simulink model "VTOL_v2"  (R2019b)
settings: Solver=FixedStepAuto  StartTime=0.0  StopTime=inf  FixedStep=Ts  RelTol=1e-3  EnableMultiTasking=on
values from neighbouring files (symbols this model uses):
  k1 = (0.5/axisgains(2) - k2*cruiseThrottle^2)/(cruiseVel^2)    [SensitivityParameterFinder.m]
  k2 = 0.5/(axisgains(2)*hoverpower(1).^2)    [SensitivityParameterFinder.m]
  k3 = (0.5/axisgains(1) - k4*cruiseThrottle^2)/(cruiseVel^2)    [SensitivityParameterFinder.m]
  k4 = 0.5/(axisgains(1)*hoverpower(1).^2)    [SensitivityParameterFinder.m]
  Ts = 1/100    (= 0.01)    [VTOL_params.m]
undefined symbols (not defined in the file or in its folder): color, deltaprops, dev, led_mask, Main, mode, MRC, pwm_output0
libraries: px4uORBlib x13, aerolibutil x8, simulink x6, pwm_sig_converters x4, px4Sensorslib x2, px4lib x2, sharedtransform x2
(part 2 of 3)

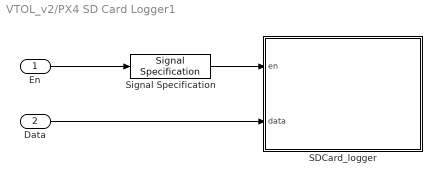
== system VTOL_v2/PX4 SD Card Logger1 ==
  En : Inport
  Data : Inport  Port=2
  SDCard_logger : MATLAB Function  TreatAsAtomicUnit=on
  Signal Specification : SignalSpecification  OutDataTypeStr=boolean
  wires:
  Signal Specification/1 -> SDCard_logger/1(en)
  En/1 -> Signal Specification/1
  Data/1 -> SDCard_logger/2(data)

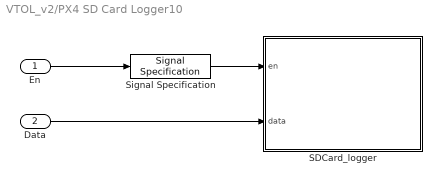
== system VTOL_v2/PX4 SD Card Logger10 ==
  En : Inport
  Data : Inport  Port=2
  SDCard_logger : MATLAB Function  TreatAsAtomicUnit=on
  Signal Specification : SignalSpecification  OutDataTypeStr=boolean
  wires:
  Signal Specification/1 -> SDCard_logger/1(en)
  En/1 -> Signal Specification/1
  Data/1 -> SDCard_logger/2(data)

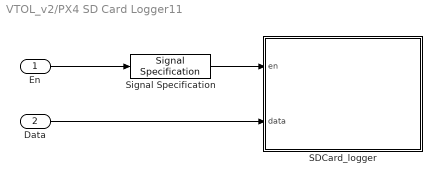
== system VTOL_v2/PX4 SD Card Logger11 ==
  En : Inport
  Data : Inport  Port=2
  SDCard_logger : MATLAB Function  TreatAsAtomicUnit=on
  Signal Specification : SignalSpecification  OutDataTypeStr=boolean
  wires:
  Signal Specification/1 -> SDCard_logger/1(en)
  En/1 -> Signal Specification/1
  Data/1 -> SDCard_logger/2(data)

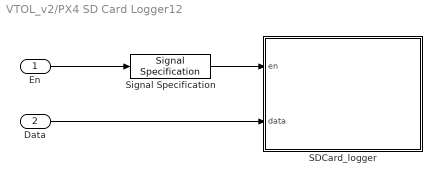
== system VTOL_v2/PX4 SD Card Logger12 ==
  En : Inport
  Data : Inport  Port=2
  SDCard_logger : MATLAB Function  TreatAsAtomicUnit=on
  Signal Specification : SignalSpecification  OutDataTypeStr=boolean
  wires:
  Signal Specification/1 -> SDCard_logger/1(en)
  En/1 -> Signal Specification/1
  Data/1 -> SDCard_logger/2(data)

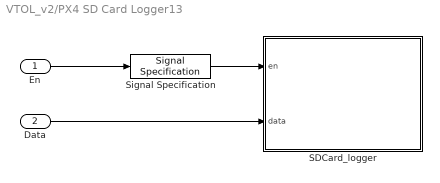
== system VTOL_v2/PX4 SD Card Logger13 ==
  En : Inport
  Data : Inport  Port=2
  SDCard_logger : MATLAB Function  TreatAsAtomicUnit=on
  Signal Specification : SignalSpecification  OutDataTypeStr=boolean
  wires:
  Signal Specification/1 -> SDCard_logger/1(en)
  En/1 -> Signal Specification/1
  Data/1 -> SDCard_logger/2(data)

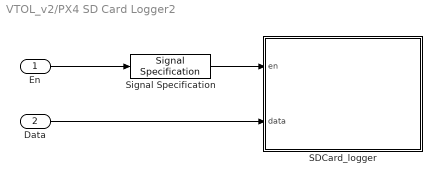
== system VTOL_v2/PX4 SD Card Logger2 ==
  En : Inport
  Data : Inport  Port=2
  SDCard_logger : MATLAB Function  TreatAsAtomicUnit=on
  Signal Specification : SignalSpecification  OutDataTypeStr=boolean
  wires:
  Signal Specification/1 -> SDCard_logger/1(en)
  En/1 -> Signal Specification/1
  Data/1 -> SDCard_logger/2(data)

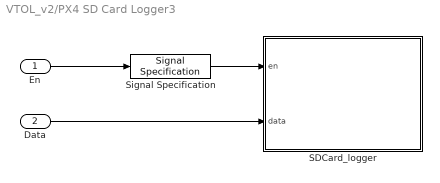
== system VTOL_v2/PX4 SD Card Logger3 ==
  En : Inport
  Data : Inport  Port=2
  SDCard_logger : MATLAB Function  TreatAsAtomicUnit=on
  Signal Specification : SignalSpecification  OutDataTypeStr=boolean
  wires:
  Signal Specification/1 -> SDCard_logger/1(en)
  En/1 -> Signal Specification/1
  Data/1 -> SDCard_logger/2(data)

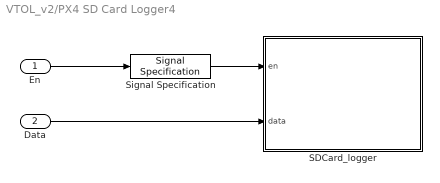
== system VTOL_v2/PX4 SD Card Logger4 ==
  En : Inport
  Data : Inport  Port=2
  SDCard_logger : MATLAB Function  TreatAsAtomicUnit=on
  Signal Specification : SignalSpecification  OutDataTypeStr=boolean
  wires:
  Signal Specification/1 -> SDCard_logger/1(en)
  En/1 -> Signal Specification/1
  Data/1 -> SDCard_logger/2(data)

== system VTOL_v2/PX4 SD Card Logger5 ==
  En : Inport
  Data : Inport  Port=2
  SDCard_logger : MATLAB Function  TreatAsAtomicUnit=on
  Signal Specification : SignalSpecification  OutDataTypeStr=boolean
  wires:
  Signal Specification/1 -> SDCard_logger/1(en)
  En/1 -> Signal Specification/1
  Data/1 -> SDCard_logger/2(data)

== system VTOL_v2/PX4 SD Card Logger6 ==
  En : Inport
  Data : Inport  Port=2
  SDCard_logger : MATLAB Function  TreatAsAtomicUnit=on
  Signal Specification : SignalSpecification  OutDataTypeStr=boolean
  wires:
  Signal Specification/1 -> SDCard_logger/1(en)
  En/1 -> Signal Specification/1
  Data/1 -> SDCard_logger/2(data)

== system VTOL_v2/PX4 SD Card Logger7 ==
  En : Inport
  Data : Inport  Port=2
  SDCard_logger : MATLAB Function  TreatAsAtomicUnit=on
  Signal Specification : SignalSpecification  OutDataTypeStr=boolean
  wires:
  Signal Specification/1 -> SDCard_logger/1(en)
  En/1 -> Signal Specification/1
  Data/1 -> SDCard_logger/2(data)

== system VTOL_v2/PX4 SD Card Logger8 ==
  En : Inport
  Data : Inport  Port=2
  SDCard_logger : MATLAB Function  TreatAsAtomicUnit=on
  Signal Specification : SignalSpecification  OutDataTypeStr=boolean
  wires:
  Signal Specification/1 -> SDCard_logger/1(en)
  En/1 -> Signal Specification/1
  Data/1 -> SDCard_logger/2(data)

== system VTOL_v2/PX4 SD Card Logger9 ==
  En : Inport
  Data : Inport  Port=2
  SDCard_logger : MATLAB Function  TreatAsAtomicUnit=on
  Signal Specification : SignalSpecification  OutDataTypeStr=boolean
  wires:
  Signal Specification/1 -> SDCard_logger/1(en)
  En/1 -> Signal Specification/1
  Data/1 -> SDCard_logger/2(data)

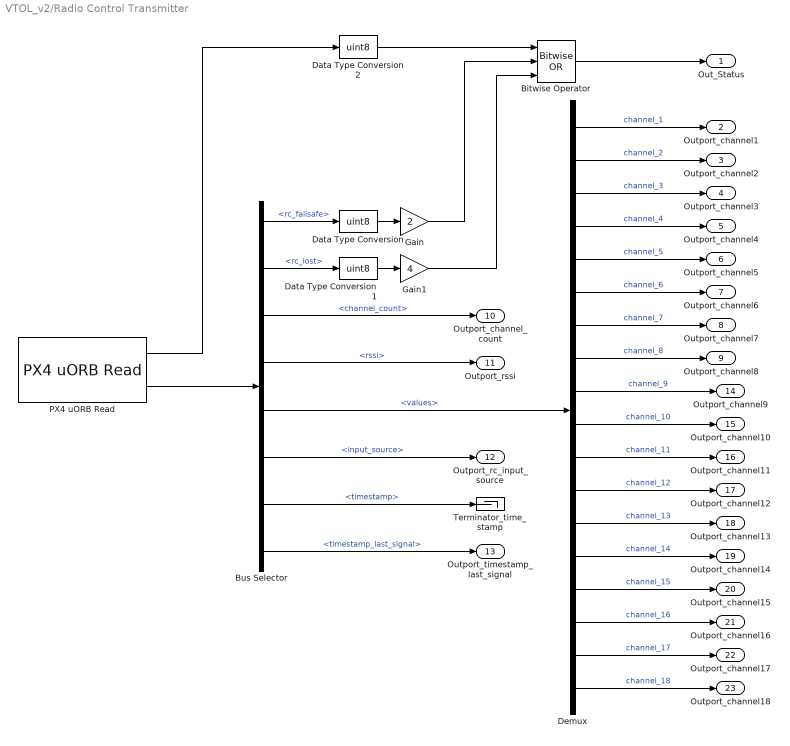
== system VTOL_v2/Radio Control Transmitter ==
  Bitwise Operator : simulink/Logic and Bit Operations/Bitwise Operator  logicop=OR  UseBitMask=off  NumInputPorts=3  BitMask=bin2dec('11011001')  BitMaskRealWorld=Stored Integer
  Bus Selector : BusSelector  OutputSignals=rc_failsafe,rc_lost,channel_count,rssi,values,input_source,timestamp,timestamp_last_signal
  Data Type Conversion : DataTypeConversion  OutDataTypeStr=uint8
  Data Type Conversion1 : DataTypeConversion  OutDataTypeStr=uint8
  Data Type Conversion2 : DataTypeConversion  OutDataTypeStr=uint8
  Demux : Demux  Outputs=18
  Gain : Gain  Gain=2  OutDataTypeStr=uint8
  Gain1 : Gain  Gain=4  OutDataTypeStr=uint8
  PX4 uORB Read : px4uORBlib/PX4 uORB Read  uORBTopic=input_rc  sampleTime=sampleTime  BlockingMode=off  BlockTimeout=BlockTimeout
      settings: SourceProductName=Embedded Coder Support Package for PX4 Autopilots  SourceProductBaseCode=PX4AUTOPILOTS
  Terminator_time_stamp : Terminator
  Out_Status : Outport  VectorParamsAs1DForOutWhenUnconnected=off
  Outport_channel1 : Outport  Port=2  VectorParamsAs1DForOutWhenUnconnected=off
  Outport_channel2 : Outport  Port=3  VectorParamsAs1DForOutWhenUnconnected=off
  Outport_channel3 : Outport  Port=4  VectorParamsAs1DForOutWhenUnconnected=off
  Outport_channel4 : Outport  Port=5  VectorParamsAs1DForOutWhenUnconnected=off
  Outport_channel5 : Outport  Port=6
  Outport_channel6 : Outport  Port=7
  Outport_channel7 : Outport  Port=8
  Outport_channel8 : Outport  Port=9
  Outport_channel_count : Outport  Port=10
  Outport_rssi : Outport  Port=11
  Outport_rc_input_source : Outport  Port=12
  Outport_timestamp_last_signal : Outport  Port=13
  Outport_channel9 : Outport  Port=14  VectorParamsAs1DForOutWhenUnconnected=off
  Outport_channel10 : Outport  Port=15  VectorParamsAs1DForOutWhenUnconnected=off
  Outport_channel11 : Outport  Port=16  VectorParamsAs1DForOutWhenUnconnected=off
  Outport_channel12 : Outport  Port=17  VectorParamsAs1DForOutWhenUnconnected=off
  Outport_channel13 : Outport  Port=18
  Outport_channel14 : Outport  Port=19
  Outport_channel15 : Outport  Port=20
  Outport_channel16 : Outport  Port=21
  Outport_channel17 : Outport  Port=22
  Outport_channel18 : Outport  Port=23
  wires:
  Data Type Conversion2/1 -> Bitwise Operator/1
  Gain1/1 -> Bitwise Operator/3
  Gain/1 -> Bitwise Operator/2
  PX4 uORB Read/1 -> Data Type Conversion2/1
  Bitwise Operator/1 -> Out_Status/1
  Data Type Conversion1/1 -> Gain1/1
  Data Type Conversion/1 -> Gain/1
  Bus Selector/8 -> Outport_timestamp_last_signal/1  "<timestamp_last_signal>"
  Demux/11 -> Outport_channel11/1  "channel_11"
  Demux/3 -> Outport_channel3/1  "channel_3"
  Demux/16 -> Outport_channel16/1  "channel_16"
  Demux/13 -> Outport_channel13/1  "channel_13"
  Demux/18 -> Outport_channel18/1  "channel_18"
  Demux/15 -> Outport_channel15/1  "channel_15"
  Bus Selector/3 -> Outport_channel_count/1  "<channel_count>"
  Demux/17 -> Outport_channel17/1  "channel_17"
  Demux/9 -> Outport_channel9/1  "channel_9"
  Bus Selector/5 -> Demux/1  "<values>"
  Bus Selector/6 -> Outport_rc_input_source/1  "<input_source>"
  Demux/10 -> Outport_channel10/1  "channel_10"
  Demux/1 -> Outport_channel1/1  "channel_1"
  Demux/12 -> Outport_channel12/1  "channel_12"
  Demux/14 -> Outport_channel14/1  "channel_14"
  Demux/6 -> Outport_channel6/1  "channel_6"
  PX4 uORB Read/2 -> Bus Selector/1
  Demux/5 -> Outport_channel5/1  "channel_5"
  Demux/7 -> Outport_channel7/1  "channel_7"
  Demux/2 -> Outport_channel2/1  "channel_2"
  Demux/8 -> Outport_channel8/1  "channel_8"
  Demux/4 -> Outport_channel4/1  "channel_4"
  Bus Selector/4 -> Outport_rssi/1  "<rssi>"
  Bus Selector/1 -> Data Type Conversion/1  "<rc_failsafe>"
  Bus Selector/2 -> Data Type Conversion1/1  "<rc_lost>"
  Bus Selector/7 -> Terminator_time_stamp/1  "<timestamp>"

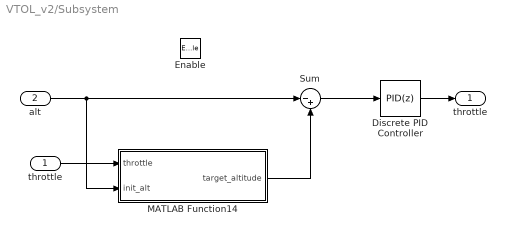
== system VTOL_v2/Subsystem ==
  throttle : Inport
  alt : Inport  Port=2
  Enable : EnablePort  StatesWhenEnabling=reset
  Discrete PID Controller : simulink/Continuous/PID Controller  Controller=PID  Form=Parallel  TimeDomain=Discrete-time  SampleTime=-1  IntegratorMethod=Forward Euler  FilterMethod=Forward Euler  ControllerParametersSource=internal  P=0.5  I=0.03  D=0.1  UseFilter=off  N=100  TunerSelectOption=Transfer Function Based (PID Tuner App)  InitialConditionSource=internal  InitialConditionForIntegrator=0  InitialConditionForFilter=0  DifferentiatorICPrevScaledInput=0  ExternalReset=none  TrackingMode=off  Kt=1  LimitOutput=on  UpperSaturationLimit=1  LowerSaturationLimit=-1  LinearizeAsGain=off  AntiWindupMode=none  Kb=1  POutMin=[]  POutMax=[]  IOutMin=[]  IOutMax=[]  DOutMin=[]  DOutMax=[]  NOutMin=[]  NOutMax=[]  SumOutMin=[]  SumOutMax=[]  SaturationOutMin=[]  SaturationOutMax=[]  PParamMin=[]  PParamMax=[]  IParamMin=[]  IParamMax=[]  DParamMin=[]  DParamMax=[]  NParamMin=[]  NParamMax=[]  KbParamMin=[]  KbParamMax=[]  KtParamMin=[]  KtParamMax=[]  KbOutMin=[]  KbOutMax=[]  KtOutMin=[]  KtOutMax=[]  IntegratorOutMin=[]  IntegratorOutMax=[]  FilterOutMin=[]  FilterOutMax=[]  SumI1OutMin=[]  SumI1OutMax=[]  SumI2OutMin=[]  SumI2OutMax=[]  SumI3OutMin=[]  SumI3OutMax=[]  SumI4OutMin=[]  SumI4OutMax=[]  SumDOutMin=[]  SumDOutMax=[]  DifferentiatorOutMin=[]  DifferentiatorOutMax=[]  FilterDiffOutCoefMin=[]  FilterDiffOutCoefMax=[]  ReciprocalOutMin=[]  ReciprocalOutMax=[]  SumDenOutMin=[]  SumDenOutMax=[]  SumNumOutMin=[]  SumNumOutMax=[]  DivideOutMin=[]  DivideOutMax=[]  IntegratorContinuousStateAttributes=''  IntegratorStateMustResolveToSignalObject=off  IntegratorRTWStateStorageClass=Auto  FilterContinuousStateAttributes=''  FilterStateMustResolveToSignalObject=off  FilterRTWStateStorageClass=Auto  ParallelPVariant=InternalParameters  IdealPVariant=Disabled  IVariant=InternalParameters  DVariant=InternalParameters  IntegratorVariant=Discrete  SatVariant=Enabled  AWVariant=Passthrough  PCopyVariant=Disabled  TRVariant=Disabled  FdbkBlocksVariant=Forward  IdealPFdbkVariant=Disabled  SatFdbkVariant=Disabled  DerivativeFilterVariant=Differentiator  NVariant=Passthrough  NCopyVariant=Disabled_SignalSpec  FilterICVariant=InternalICsDifferentiator  IntegratorICVariant=InternalICs  ExternalResetVariant=Disabled  TRSumVariant=Passthrough  SumFdbkVariant=Disabled  SumVariant=Sum_PID
  MATLAB Function14 : MATLAB Function  TreatAsAtomicUnit=on
  Sum : Sum  Inputs=|-+
  "throttle " : Outport  VectorParamsAs1DForOutWhenUnconnected=off
  wires:
  throttle/1 -> MATLAB Function14/1(throttle)
  MATLAB Function14/1(target_altitude) -> Sum/2
  Sum/1 -> Discrete PID Controller/1
  Discrete PID Controller/1 -> "throttle "/1
  alt/1 -> MATLAB Function14/2(init_alt), Sum/1

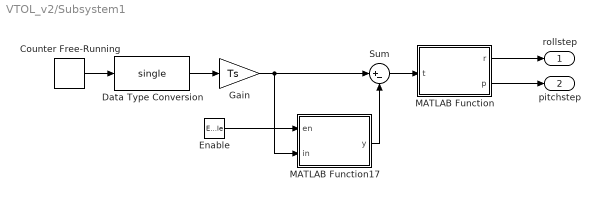
== system VTOL_v2/Subsystem1 ==
  Enable : EnablePort  StatesWhenEnabling=reset  ShowOutputPort=on
  Counter Free-Running : simulink/Sources/Counter Free-Running  NumBits=16  tsamp=Ts
  Data Type Conversion : DataTypeConversion  OutDataTypeStr=single
  Gain : Gain  Gain=Ts
  MATLAB Function : MATLAB Function  TreatAsAtomicUnit=on
  MATLAB Function17 : MATLAB Function  TreatAsAtomicUnit=on
  Sum : Sum  Inputs=|+-
  rollstep : Outport
  pitchstep : Outport  Port=2
  wires:
  Enable/1 -> MATLAB Function17/1(en)
  Data Type Conversion/1 -> Gain/1
  MATLAB Function17/1(y) -> Sum/2
  Sum/1 -> MATLAB Function/1(t)
  MATLAB Function/1(r) -> rollstep/1
  MATLAB Function/2(p) -> pitchstep/1
  Counter Free-Running/1 -> Data Type Conversion/1
  Gain/1 -> MATLAB Function17/2(in), Sum/1

== matlab function VTOL_v2/PX4 SD Card Logger10/SDCard_logger ==
  data: en input boolean; data input; logname parameter uint8; cacheflag parameter boolean; numRecs parameter uint32
%% PX4 SD Card Logger
% Note: All data needs to be of the same type (e.g. double)
% Header information format:
%           String "MWLOG"
%           Time/Date 4 bytes (time())
%           Number of Signals per record Logged 1 byte (256 max)
%           Data Type of Signals Logged  1 byte (1-10)
%           Number of bytes per record 2 bytes (65535 max)
% This does NOT include the number of data sets logged.
% i.e. The Reader is responsible for reading until EOF.
% Steve Kuznicki
% Copyright 2018 The MathWorks, Inc.

function SDCard_logger(en, data, logname, cacheflag, numRecs)

persistent fp count elem_size vect_size datastore timestore count_prev

if coder.target('Rtw')
    
    coder.cinclude('<stdio.h>');
    coder.cinclude('<time.h>');
    
    if coder.target('Rtw')
        coder.cinclude('<drivers/drv_hrt.h>');
    end
    
    if coder.target('Rtw')
        timestamp=coder.opaque('uint64_t');
        timestamp=coder.ceval('hrt_absolute_time');
    else
        timestamp = uint64(0);
    end
    
    if isempty(count)
        count = uint32(0);
        count_prev=count;
        fp = coder.opaque('FILE*', 'NULL');
        if cacheflag == true
            datastore = zeros(numRecs*uint32(coder.const(numel(data))), 1, 'like', data);
            timestore=uint64(zeros(numRecs, 1));
        end
        
        [elsize, eltype] = get_elem_size(data);
        elem_size = coder.const(uint16(elsize));
        elem_type = coder.const(uint8(eltype));
        vect_size = coder.const(uint8(numel(data)));
        coder.ceval('printf',['OPENING file %s vect_size %d elem_size %d numRecs %d %c' uint8(0)], ...
            [logname,'.bin', int8(0)], uint32(vect_size), uint32(elem_size), uint32(numRecs), uint8(10));
        fp = coder.ceval('fopen', [logname,'.bin', int8(0)], ['wb', int8(0)]);
        
        % Write header information here
        % header token + version
        mlStrVer = 'MWLOG';
        coder.ceval('fwrite', coder.rref(mlStrVer), uint32(1), length(mlStrVer), fp);
        % date/time
        tm = uint32(0);
        tmptr = uint32(0);
        tm = coder.ceval('time',coder.wref(tmptr));
        coder.ceval('fwrite', coder.rref(tm), uint32(4), uint32(1), fp);
        % number of elements in each record
        coder.ceval('fwrite', coder.rref(vect_size), uint32(1), uint32(1), fp);
        % data type of the elements
        coder.ceval('fwrite', coder.rref(elem_type), uint32(1), uint32(1), fp);
        % size of each record in bytes
        recSize = elem_size * uint16(vect_size);
        coder.ceval('fwrite', coder.rref(recSize), uint32(2), uint32(1), fp);
        coder.ceval('fclose', fp);
    end
    
    
    if (en && (count < numRecs))
              
        % cache data in memory or use fwrite
        if cacheflag == true
            addr = (count*uint32(vect_size))+1;
            for idx = 1:vect_size
                datastore(addr) = data(idx);
                addr = addr + 1;
            end
            timestore(count+uint32(1))=uint64(timestamp);
        else
            % open file in append mode
            fp = coder.ceval('fopen', [logname,'.bin', int8(0)], ['ab', int8(0)]);
            coder.ceval('fwrite', coder.rref(data), elem_size, vect_size, fp);
            if coder.target('Rtw')
                coder.ceval('fwrite', coder.rref(timestamp), uint32(8), uint32(1), fp);
            end
            coder.ceval('fflush', fp);
            coder.ceval('fclose', fp);
        end
        count = count + uint32(1);
        
    else
        
        if cacheflag
            % open file in append mode
            fp = coder.ceval('fopen', [logname,'.bin', int8(0)], ['ab', int8(0)]);
            coder.ceval('printf',['CLOSING file. count = %d %c' uint8(0)], uint32(count), uint8(10));
            for idx=count_prev+1:count
                for idx2=(idx-1)*double(vect_size)+1:(idx-1)*double(vect_size)+double(vect_size)
                    coder.ceval('fwrite', coder.rref(datastore(idx2)), elem_size, uint32(1), fp);
                end
                coder.ceval('fwrite', coder.rref(timestore(idx)), uint32(8), uint32(1), fp);
            end
            coder.ceval('fflush', fp);
            coder.ceval('fclose', fp);
        end
        count_prev=count;
    end
end

% return the size of the element in bytes
    function [elem_size, dtype] = get_elem_size(data)
        switch(class(data))
            case 'double'
                elem_size = 8;
                dtype = 1;
            case 'single'
                elem_size = 4;
                dtype = 2;
            case 'int32'
                elem_size = 4;
                dtype = 3;
            case 'uint32'
                elem_size = 4;
                dtype = 4;
            case 'int16'
                elem_size = 2;
                dtype = 5;
            case 'uint16'
                elem_size = 2;
                dtype = 6;
            case 'int8'
                elem_size = 1;
                dtype = 7;
            case 'uint8'
                elem_size = 1;
                dtype = 8;
            case 'logical'
                elem_size = 1;
                dtype = 9;
            case 'embedded.fi'
                nt = numerictype(data);
                elem_size = 2^ceil(log2(ceil(nt.WordLength / 8)));
                dtype = 10;
        end
        if ~isreal(data)
            elem_size = elem_size*2;
        end
        
        elem_size = uint16(elem_size);
        dtype = uint8(dtype);
    end
end

== matlab function VTOL_v2/PX4 SD Card Logger11/SDCard_logger ==
  data: en input boolean; data input; logname parameter uint8; cacheflag parameter boolean; numRecs parameter uint32
%% PX4 SD Card Logger
% Note: All data needs to be of the same type (e.g. double)
% Header information format:
%           String "MWLOG"
%           Time/Date 4 bytes (time())
%           Number of Signals per record Logged 1 byte (256 max)
%           Data Type of Signals Logged  1 byte (1-10)
%           Number of bytes per record 2 bytes (65535 max)
% This does NOT include the number of data sets logged.
% i.e. The Reader is responsible for reading until EOF.
% Steve Kuznicki
% Copyright 2018 The MathWorks, Inc.

function SDCard_logger(en, data, logname, cacheflag, numRecs)

persistent fp count elem_size vect_size datastore timestore count_prev

if coder.target('Rtw')
    
    coder.cinclude('<stdio.h>');
    coder.cinclude('<time.h>');
    
    if coder.target('Rtw')
        coder.cinclude('<drivers/drv_hrt.h>');
    end
    
    if coder.target('Rtw')
        timestamp=coder.opaque('uint64_t');
        timestamp=coder.ceval('hrt_absolute_time');
    else
        timestamp = uint64(0);
    end
    
    if isempty(count)
        count = uint32(0);
        count_prev=count;
        fp = coder.opaque('FILE*', 'NULL');
        if cacheflag == true
            datastore = zeros(numRecs*uint32(coder.const(numel(data))), 1, 'like', data);
            timestore=uint64(zeros(numRecs, 1));
        end
        
        [elsize, eltype] = get_elem_size(data);
        elem_size = coder.const(uint16(elsize));
        elem_type = coder.const(uint8(eltype));
        vect_size = coder.const(uint8(numel(data)));
        coder.ceval('printf',['OPENING file %s vect_size %d elem_size %d numRecs %d %c' uint8(0)], ...
            [logname,'.bin', int8(0)], uint32(vect_size), uint32(elem_size), uint32(numRecs), uint8(10));
        fp = coder.ceval('fopen', [logname,'.bin', int8(0)], ['wb', int8(0)]);
        
        % Write header information here
        % header token + version
        mlStrVer = 'MWLOG';
        coder.ceval('fwrite', coder.rref(mlStrVer), uint32(1), length(mlStrVer), fp);
        % date/time
        tm = uint32(0);
        tmptr = uint32(0);
        tm = coder.ceval('time',coder.wref(tmptr));
        coder.ceval('fwrite', coder.rref(tm), uint32(4), uint32(1), fp);
        % number of elements in each record
        coder.ceval('fwrite', coder.rref(vect_size), uint32(1), uint32(1), fp);
        % data type of the elements
        coder.ceval('fwrite', coder.rref(elem_type), uint32(1), uint32(1), fp);
        % size of each record in bytes
        recSize = elem_size * uint16(vect_size);
        coder.ceval('fwrite', coder.rref(recSize), uint32(2), uint32(1), fp);
        coder.ceval('fclose', fp);
    end
    
    
    if (en && (count < numRecs))
              
        % cache data in memory or use fwrite
        if cacheflag == true
            addr = (count*uint32(vect_size))+1;
            for idx = 1:vect_size
                datastore(addr) = data(idx);
                addr = addr + 1;
            end
            timestore(count+uint32(1))=uint64(timestamp);
        else
            % open file in append mode
            fp = coder.ceval('fopen', [logname,'.bin', int8(0)], ['ab', int8(0)]);
            coder.ceval('fwrite', coder.rref(data), elem_size, vect_size, fp);
            if coder.target('Rtw')
                coder.ceval('fwrite', coder.rref(timestamp), uint32(8), uint32(1), fp);
            end
            coder.ceval('fflush', fp);
            coder.ceval('fclose', fp);
        end
        count = count + uint32(1);
        
    else
        
        if cacheflag
            % open file in append mode
            fp = coder.ceval('fopen', [logname,'.bin', int8(0)], ['ab', int8(0)]);
            coder.ceval('printf',['CLOSING file. count = %d %c' uint8(0)], uint32(count), uint8(10));
            for idx=count_prev+1:count
                for idx2=(idx-1)*double(vect_size)+1:(idx-1)*double(vect_size)+double(vect_size)
                    coder.ceval('fwrite', coder.rref(datastore(idx2)), elem_size, uint32(1), fp);
                end
                coder.ceval('fwrite', coder.rref(timestore(idx)), uint32(8), uint32(1), fp);
            end
            coder.ceval('fflush', fp);
            coder.ceval('fclose', fp);
        end
        count_prev=count;
    end
end

% return the size of the element in bytes
    function [elem_size, dtype] = get_elem_size(data)
        switch(class(data))
            case 'double'
                elem_size = 8;
                dtype = 1;
            case 'single'
                elem_size = 4;
                dtype = 2;
            case 'int32'
                elem_size = 4;
                dtype = 3;
            case 'uint32'
                elem_size = 4;
                dtype = 4;
            case 'int16'
                elem_size = 2;
                dtype = 5;
            case 'uint16'
                elem_size = 2;
                dtype = 6;
            case 'int8'
                elem_size = 1;
                dtype = 7;
            case 'uint8'
                elem_size = 1;
                dtype = 8;
            case 'logical'
                elem_size = 1;
                dtype = 9;
            case 'embedded.fi'
                nt = numerictype(data);
                elem_size = 2^ceil(log2(ceil(nt.WordLength / 8)));
                dtype = 10;
        end
        if ~isreal(data)
            elem_size = elem_size*2;
        end
        
        elem_size = uint16(elem_size);
        dtype = uint8(dtype);
    end
end

== matlab function VTOL_v2/PX4 SD Card Logger12/SDCard_logger ==
  data: en input boolean; data input; logname parameter uint8; cacheflag parameter boolean; numRecs parameter uint32
%% PX4 SD Card Logger
% Note: All data needs to be of the same type (e.g. double)
% Header information format:
%           String "MWLOG"
%           Time/Date 4 bytes (time())
%           Number of Signals per record Logged 1 byte (256 max)
%           Data Type of Signals Logged  1 byte (1-10)
%           Number of bytes per record 2 bytes (65535 max)
% This does NOT include the number of data sets logged.
% i.e. The Reader is responsible for reading until EOF.
% Steve Kuznicki
% Copyright 2018 The MathWorks, Inc.

function SDCard_logger(en, data, logname, cacheflag, numRecs)

persistent fp count elem_size vect_size datastore timestore count_prev

if coder.target('Rtw')
    
    coder.cinclude('<stdio.h>');
    coder.cinclude('<time.h>');
    
    if coder.target('Rtw')
        coder.cinclude('<drivers/drv_hrt.h>');
    end
    
    if coder.target('Rtw')
        timestamp=coder.opaque('uint64_t');
        timestamp=coder.ceval('hrt_absolute_time');
    else
        timestamp = uint64(0);
    end
    
    if isempty(count)
        count = uint32(0);
        count_prev=count;
        fp = coder.opaque('FILE*', 'NULL');
        if cacheflag == true
            datastore = zeros(numRecs*uint32(coder.const(numel(data))), 1, 'like', data);
            timestore=uint64(zeros(numRecs, 1));
        end
        
        [elsize, eltype] = get_elem_size(data);
        elem_size = coder.const(uint16(elsize));
        elem_type = coder.const(uint8(eltype));
        vect_size = coder.const(uint8(numel(data)));
        coder.ceval('printf',['OPENING file %s vect_size %d elem_size %d numRecs %d %c' uint8(0)], ...
            [logname,'.bin', int8(0)], uint32(vect_size), uint32(elem_size), uint32(numRecs), uint8(10));
        fp = coder.ceval('fopen', [logname,'.bin', int8(0)], ['wb', int8(0)]);
        
        % Write header information here
        % header token + version
        mlStrVer = 'MWLOG';
        coder.ceval('fwrite', coder.rref(mlStrVer), uint32(1), length(mlStrVer), fp);
        % date/time
        tm = uint32(0);
        tmptr = uint32(0);
        tm = coder.ceval('time',coder.wref(tmptr));
        coder.ceval('fwrite', coder.rref(tm), uint32(4), uint32(1), fp);
        % number of elements in each record
        coder.ceval('fwrite', coder.rref(vect_size), uint32(1), uint32(1), fp);
        % data type of the elements
        coder.ceval('fwrite', coder.rref(elem_type), uint32(1), uint32(1), fp);
        % size of each record in bytes
        recSize = elem_size * uint16(vect_size);
        coder.ceval('fwrite', coder.rref(recSize), uint32(2), uint32(1), fp);
        coder.ceval('fclose', fp);
    end
    
    
    if (en && (count < numRecs))
              
        % cache data in memory or use fwrite
        if cacheflag == true
            addr = (count*uint32(vect_size))+1;
            for idx = 1:vect_size
                datastore(addr) = data(idx);
                addr = addr + 1;
            end
            timestore(count+uint32(1))=uint64(timestamp);
        else
            % open file in append mode
            fp = coder.ceval('fopen', [logname,'.bin', int8(0)], ['ab', int8(0)]);
            coder.ceval('fwrite', coder.rref(data), elem_size, vect_size, fp);
            if coder.target('Rtw')
                coder.ceval('fwrite', coder.rref(timestamp), uint32(8), uint32(1), fp);
            end
            coder.ceval('fflush', fp);
            coder.ceval('fclose', fp);
        end
        count = count + uint32(1);
        
    else
        
        if cacheflag
            % open file in append mode
            fp = coder.ceval('fopen', [logname,'.bin', int8(0)], ['ab', int8(0)]);
            coder.ceval('printf',['CLOSING file. count = %d %c' uint8(0)], uint32(count), uint8(10));
            for idx=count_prev+1:count
                for idx2=(idx-1)*double(vect_size)+1:(idx-1)*double(vect_size)+double(vect_size)
                    coder.ceval('fwrite', coder.rref(datastore(idx2)), elem_size, uint32(1), fp);
                end
                coder.ceval('fwrite', coder.rref(timestore(idx)), uint32(8), uint32(1), fp);
            end
            coder.ceval('fflush', fp);
            coder.ceval('fclose', fp);
        end
        count_prev=count;
    end
end

% return the size of the element in bytes
    function [elem_size, dtype] = get_elem_size(data)
        switch(class(data))
            case 'double'
                elem_size = 8;
                dtype = 1;
            case 'single'
                elem_size = 4;
                dtype = 2;
            case 'int32'
                elem_size = 4;
                dtype = 3;
            case 'uint32'
                elem_size = 4;
                dtype = 4;
            case 'int16'
                elem_size = 2;
                dtype = 5;
            case 'uint16'
                elem_size = 2;
                dtype = 6;
            case 'int8'
                elem_size = 1;
                dtype = 7;
            case 'uint8'
                elem_size = 1;
                dtype = 8;
            case 'logical'
                elem_size = 1;
                dtype = 9;
            case 'embedded.fi'
                nt = numerictype(data);
                elem_size = 2^ceil(log2(ceil(nt.WordLength / 8)));
                dtype = 10;
        end
        if ~isreal(data)
            elem_size = elem_size*2;
        end
        
        elem_size = uint16(elem_size);
        dtype = uint8(dtype);
    end
end

== matlab function VTOL_v2/PX4 SD Card Logger7/SDCard_logger ==
  data: en input boolean; data input; logname parameter uint8; cacheflag parameter boolean; numRecs parameter uint32
%% PX4 SD Card Logger
% Note: All data needs to be of the same type (e.g. double)
% Header information format:
%           String "MWLOG"
%           Time/Date 4 bytes (time())
%           Number of Signals per record Logged 1 byte (256 max)
%           Data Type of Signals Logged  1 byte (1-10)
%           Number of bytes per record 2 bytes (65535 max)
% This does NOT include the number of data sets logged.
% i.e. The Reader is responsible for reading until EOF.
% Steve Kuznicki
% Copyright 2018 The MathWorks, Inc.

function SDCard_logger(en, data, logname, cacheflag, numRecs)

persistent fp count elem_size vect_size datastore timestore count_prev

if coder.target('Rtw')
    
    coder.cinclude('<stdio.h>');
    coder.cinclude('<time.h>');
    
    if coder.target('Rtw')
        coder.cinclude('<drivers/drv_hrt.h>');
    end
    
    if coder.target('Rtw')
        timestamp=coder.opaque('uint64_t');
        timestamp=coder.ceval('hrt_absolute_time');
    else
        timestamp = uint64(0);
    end
    
    if isempty(count)
        count = uint32(0);
        count_prev=count;
        fp = coder.opaque('FILE*', 'NULL');
        if cacheflag == true
            datastore = zeros(numRecs*uint32(coder.const(numel(data))), 1, 'like', data);
            timestore=uint64(zeros(numRecs, 1));
        end
        
        [elsize, eltype] = get_elem_size(data);
        elem_size = coder.const(uint16(elsize));
        elem_type = coder.const(uint8(eltype));
        vect_size = coder.const(uint8(numel(data)));
        coder.ceval('printf',['OPENING file %s vect_size %d elem_size %d numRecs %d %c' uint8(0)], ...
            [logname,'.bin', int8(0)], uint32(vect_size), uint32(elem_size), uint32(numRecs), uint8(10));
        fp = coder.ceval('fopen', [logname,'.bin', int8(0)], ['wb', int8(0)]);
        
        % Write header information here
        % header token + version
        mlStrVer = 'MWLOG';
        coder.ceval('fwrite', coder.rref(mlStrVer), uint32(1), length(mlStrVer), fp);
        % date/time
        tm = uint32(0);
        tmptr = uint32(0);
        tm = coder.ceval('time',coder.wref(tmptr));
        coder.ceval('fwrite', coder.rref(tm), uint32(4), uint32(1), fp);
        % number of elements in each record
        coder.ceval('fwrite', coder.rref(vect_size), uint32(1), uint32(1), fp);
        % data type of the elements
        coder.ceval('fwrite', coder.rref(elem_type), uint32(1), uint32(1), fp);
        % size of each record in bytes
        recSize = elem_size * uint16(vect_size);
        coder.ceval('fwrite', coder.rref(recSize), uint32(2), uint32(1), fp);
        coder.ceval('fclose', fp);
    end
    
    
    if (en && (count < numRecs))
              
        % cache data in memory or use fwrite
        if cacheflag == true
            addr = (count*uint32(vect_size))+1;
            for idx = 1:vect_size
                datastore(addr) = data(idx);
                addr = addr + 1;
            end
            timestore(count+uint32(1))=uint64(timestamp);
        else
            % open file in append mode
            fp = coder.ceval('fopen', [logname,'.bin', int8(0)], ['ab', int8(0)]);
            coder.ceval('fwrite', coder.rref(data), elem_size, vect_size, fp);
            if coder.target('Rtw')
                coder.ceval('fwrite', coder.rref(timestamp), uint32(8), uint32(1), fp);
            end
            coder.ceval('fflush', fp);
            coder.ceval('fclose', fp);
        end
        count = count + uint32(1);
        
   else
        
        if cacheflag
            % open file in append mode
            fp = coder.ceval('fopen', [logname,'.bin', int8(0)], ['ab', int8(0)]);
            coder.ceval('printf',['CLOSING file. count = %d %c' uint8(0)], uint32(count), uint8(10));
            for idx=count_prev+1:count
                for idx2=(idx-1)*double(vect_size)+1:(idx-1)*double(vect_size)+double(vect_size)
                    coder.ceval('fwrite', coder.rref(datastore(idx2)), elem_size, uint32(1), fp);
                end
                coder.ceval('fwrite', coder.rref(timestore(idx)), uint32(8), uint32(1), fp);
            end
            coder.ceval('fflush', fp);
            coder.ceval('fclose', fp);
        end
        count_prev=count;
    end
end

% return the size of the element in bytes
    function [elem_size, dtype] = get_elem_size(data)
        switch(class(data))
            case 'double'
                elem_size = 8;
                dtype = 1;
            case 'single'
                elem_size = 4;
                dtype = 2;
            case 'int32'
                elem_size = 4;
                dtype = 3;
            case 'uint32'
                elem_size = 4;
                dtype = 4;
            case 'int16'
                elem_size = 2;
                dtype = 5;
            case 'uint16'
                elem_size = 2;
                dtype = 6;
            case 'int8'
                elem_size = 1;
                dtype = 7;
            case 'uint8'
                elem_size = 1;
                dtype = 8;
            case 'logical'
                elem_size = 1;
                dtype = 9;
            case 'embedded.fi'
                nt = numerictype(data);
                elem_size = 2^ceil(log2(ceil(nt.WordLength / 8)));
                dtype = 10;
        end
        if ~isreal(data)
            elem_size = elem_size*2;
        end
        
        elem_size = uint16(elem_size);
        dtype = uint8(dtype);
    end
end

== matlab function VTOL_v2/PX4 SD Card Logger8/SDCard_logger ==
  data: en input boolean; data input; logname parameter uint8; cacheflag parameter boolean; numRecs parameter uint32
%% PX4 SD Card Logger
% Note: All data needs to be of the same type (e.g. double)
% Header information format:
%           String "MWLOG"
%           Time/Date 4 bytes (time())
%           Number of Signals per record Logged 1 byte (256 max)
%           Data Type of Signals Logged  1 byte (1-10)
%           Number of bytes per record 2 bytes (65535 max)
% This does NOT include the number of data sets logged.
% i.e. The Reader is responsible for reading until EOF.
% Steve Kuznicki
% Copyright 2018 The MathWorks, Inc.

function SDCard_logger(en, data, logname, cacheflag, numRecs)

persistent fp count elem_size vect_size datastore timestore count_prev

if coder.target('Rtw')
    
    coder.cinclude('<stdio.h>');
    coder.cinclude('<time.h>');
    
    if coder.target('Rtw')
        coder.cinclude('<drivers/drv_hrt.h>');
    end
    
    if coder.target('Rtw')
        timestamp=coder.opaque('uint64_t');
        timestamp=coder.ceval('hrt_absolute_time');
    else
        timestamp = uint64(0);
    end
    
    if isempty(count)
        count = uint32(0);
        count_prev=count;
        fp = coder.opaque('FILE*', 'NULL');
        if cacheflag == true
            datastore = zeros(numRecs*uint32(coder.const(numel(data))), 1, 'like', data);
            timestore=uint64(zeros(numRecs, 1));
        end
        
        [elsize, eltype] = get_elem_size(data);
        elem_size = coder.const(uint16(elsize));
        elem_type = coder.const(uint8(eltype));
        vect_size = coder.const(uint8(numel(data)));
        coder.ceval('printf',['OPENING file %s vect_size %d elem_size %d numRecs %d %c' uint8(0)], ...
            [logname,'.bin', int8(0)], uint32(vect_size), uint32(elem_size), uint32(numRecs), uint8(10));
        fp = coder.ceval('fopen', [logname,'.bin', int8(0)], ['wb', int8(0)]);
        
        % Write header information here
        % header token + version
        mlStrVer = 'MWLOG';
        coder.ceval('fwrite', coder.rref(mlStrVer), uint32(1), length(mlStrVer), fp);
        % date/time
        tm = uint32(0);
        tmptr = uint32(0);
        tm = coder.ceval('time',coder.wref(tmptr));
        coder.ceval('fwrite', coder.rref(tm), uint32(4), uint32(1), fp);
        % number of elements in each record
        coder.ceval('fwrite', coder.rref(vect_size), uint32(1), uint32(1), fp);
        % data type of the elements
        coder.ceval('fwrite', coder.rref(elem_type), uint32(1), uint32(1), fp);
        % size of each record in bytes
        recSize = elem_size * uint16(vect_size);
        coder.ceval('fwrite', coder.rref(recSize), uint32(2), uint32(1), fp);
        coder.ceval('fclose', fp);
    end
    
    
    if (en && (count < numRecs))
              
        % cache data in memory or use fwrite
        if cacheflag == true
            addr = (count*uint32(vect_size))+1;
            for idx = 1:vect_size
                datastore(addr) = data(idx);
                addr = addr + 1;
            end
            timestore(count+uint32(1))=uint64(timestamp);
        else
            % open file in append mode
            fp = coder.ceval('fopen', [logname,'.bin', int8(0)], ['ab', int8(0)]);
            coder.ceval('fwrite', coder.rref(data), elem_size, vect_size, fp);
            if coder.target('Rtw')
                coder.ceval('fwrite', coder.rref(timestamp), uint32(8), uint32(1), fp);
            end
            coder.ceval('fflush', fp);
            coder.ceval('fclose', fp);
        end
        count = count + uint32(1);
        
    else
        
        if cacheflag
            % open file in append mode
            fp = coder.ceval('fopen', [logname,'.bin', int8(0)], ['ab', int8(0)]);
            coder.ceval('printf',['CLOSING file. count = %d %c' uint8(0)], uint32(count), uint8(10));
            for idx=count_prev+1:count
                for idx2=(idx-1)*double(vect_size)+1:(idx-1)*double(vect_size)+double(vect_size)
                    coder.ceval('fwrite', coder.rref(datastore(idx2)), elem_size, uint32(1), fp);
                end
                coder.ceval('fwrite', coder.rref(timestore(idx)), uint32(8), uint32(1), fp);
            end
            coder.ceval('fflush', fp);
            coder.ceval('fclose', fp);
        end
        count_prev=count;
    end
end

% return the size of the element in bytes
    function [elem_size, dtype] = get_elem_size(data)
        switch(class(data))
            case 'double'
                elem_size = 8;
                dtype = 1;
            case 'single'
                elem_size = 4;
                dtype = 2;
            case 'int32'
                elem_size = 4;
                dtype = 3;
            case 'uint32'
                elem_size = 4;
                dtype = 4;
            case 'int16'
                elem_size = 2;
                dtype = 5;
            case 'uint16'
                elem_size = 2;
                dtype = 6;
            case 'int8'
                elem_size = 1;
                dtype = 7;
            case 'uint8'
                elem_size = 1;
                dtype = 8;
            case 'logical'
                elem_size = 1;
                dtype = 9;
            case 'embedded.fi'
                nt = numerictype(data);
                elem_size = 2^ceil(log2(ceil(nt.WordLength / 8)));
                dtype = 10;
        end
        if ~isreal(data)
            elem_size = elem_size*2;
        end
        
        elem_size = uint16(elem_size);
        dtype = uint8(dtype);
    end
end

== matlab function VTOL_v2/PX4 SD Card Logger9/SDCard_logger ==
  data: en input boolean; data input; logname parameter uint8; cacheflag parameter boolean; numRecs parameter uint32
%% PX4 SD Card Logger
% Note: All data needs to be of the same type (e.g. double)
% Header information format:
%           String "MWLOG"
%           Time/Date 4 bytes (time())
%           Number of Signals per record Logged 1 byte (256 max)
%           Data Type of Signals Logged  1 byte (1-10)
%           Number of bytes per record 2 bytes (65535 max)
% This does NOT include the number of data sets logged.
% i.e. The Reader is responsible for reading until EOF.
% Steve Kuznicki
% Copyright 2018 The MathWorks, Inc.

function SDCard_logger(en, data, logname, cacheflag, numRecs)

persistent fp count elem_size vect_size datastore timestore count_prev

if coder.target('Rtw')
    
    coder.cinclude('<stdio.h>');
    coder.cinclude('<time.h>');
    
    if coder.target('Rtw')
        coder.cinclude('<drivers/drv_hrt.h>');
    end
    
    if coder.target('Rtw')
        timestamp=coder.opaque('uint64_t');
        timestamp=coder.ceval('hrt_absolute_time');
    else
        timestamp = uint64(0);
    end
    
    if isempty(count)
        count = uint32(0);
        count_prev=count;
        fp = coder.opaque('FILE*', 'NULL');
        if cacheflag == true
            datastore = zeros(numRecs*uint32(coder.const(numel(data))), 1, 'like', data);
            timestore=uint64(zeros(numRecs, 1));
        end
        
        [elsize, eltype] = get_elem_size(data);
        elem_size = coder.const(uint16(elsize));
        elem_type = coder.const(uint8(eltype));
        vect_size = coder.const(uint8(numel(data)));
        coder.ceval('printf',['OPENING file %s vect_size %d elem_size %d numRecs %d %c' uint8(0)], ...
            [logname,'.bin', int8(0)], uint32(vect_size), uint32(elem_size), uint32(numRecs), uint8(10));
        fp = coder.ceval('fopen', [logname,'.bin', int8(0)], ['wb', int8(0)]);
        
        % Write header information here
        % header token + version
        mlStrVer = 'MWLOG';
        coder.ceval('fwrite', coder.rref(mlStrVer), uint32(1), length(mlStrVer), fp);
        % date/time
        tm = uint32(0);
        tmptr = uint32(0);
        tm = coder.ceval('time',coder.wref(tmptr));
        coder.ceval('fwrite', coder.rref(tm), uint32(4), uint32(1), fp);
        % number of elements in each record
        coder.ceval('fwrite', coder.rref(vect_size), uint32(1), uint32(1), fp);
        % data type of the elements
        coder.ceval('fwrite', coder.rref(elem_type), uint32(1), uint32(1), fp);
        % size of each record in bytes
        recSize = elem_size * uint16(vect_size);
        coder.ceval('fwrite', coder.rref(recSize), uint32(2), uint32(1), fp);
        coder.ceval('fclose', fp);
    end
    
    
    if (en && (count < numRecs))
              
        % cache data in memory or use fwrite
        if cacheflag == true
            addr = (count*uint32(vect_size))+1;
            for idx = 1:vect_size
                datastore(addr) = data(idx);
                addr = addr + 1;
            end
            timestore(count+uint32(1))=uint64(timestamp);
        else
            % open file in append mode
            fp = coder.ceval('fopen', [logname,'.bin', int8(0)], ['ab', int8(0)]);
            coder.ceval('fwrite', coder.rref(data), elem_size, vect_size, fp);
            if coder.target('Rtw')
                coder.ceval('fwrite', coder.rref(timestamp), uint32(8), uint32(1), fp);
            end
            coder.ceval('fflush', fp);
            coder.ceval('fclose', fp);
        end
        count = count + uint32(1);
        
    else
        
        if cacheflag
            % open file in append mode
            fp = coder.ceval('fopen', [logname,'.bin', int8(0)], ['ab', int8(0)]);
            coder.ceval('printf',['CLOSING file. count = %d %c' uint8(0)], uint32(count), uint8(10));
            for idx=count_prev+1:count
                for idx2=(idx-1)*double(vect_size)+1:(idx-1)*double(vect_size)+double(vect_size)
                    coder.ceval('fwrite', coder.rref(datastore(idx2)), elem_size, uint32(1), fp);
                end
                coder.ceval('fwrite', coder.rref(timestore(idx)), uint32(8), uint32(1), fp);
            end
            coder.ceval('fflush', fp);
            coder.ceval('fclose', fp);
        end
        count_prev=count;
    end
end

% return the size of the element in bytes
    function [elem_size, dtype] = get_elem_size(data)
        switch(class(data))
            case 'double'
                elem_size = 8;
                dtype = 1;
            case 'single'
                elem_size = 4;
                dtype = 2;
            case 'int32'
                elem_size = 4;
                dtype = 3;
            case 'uint32'
                elem_size = 4;
                dtype = 4;
            case 'int16'
                elem_size = 2;
                dtype = 5;
            case 'uint16'
                elem_size = 2;
                dtype = 6;
            case 'int8'
                elem_size = 1;
                dtype = 7;
            case 'uint8'
                elem_size = 1;
                dtype = 8;
            case 'logical'
                elem_size = 1;
                dtype = 9;
            case 'embedded.fi'
                nt = numerictype(data);
                elem_size = 2^ceil(log2(ceil(nt.WordLength / 8)));
                dtype = 10;
        end
        if ~isreal(data)
            elem_size = elem_size*2;
        end
        
        elem_size = uint16(elem_size);
        dtype = uint8(dtype);
    end
end

== matlab function VTOL_v2/MATLAB Function ==
  data: ADC input; airspeed output; zeroSignal input
function airspeed = fcn(ADC, zeroSignal)

Vs = 2*zeroSignal; % From calibration data
rho = 1.225;

% The manufacturer specifies:
% Vout = Vs*(0.2*P(kPa) + 0.5) +- 6.25% V_Fss
% So the delta P is given by:
% dP = 1000*(Vout-0.5*Vs)/(Vs*0.2) % In Pa, not kPa
% dP = 5000*(Vout/Vs - 0.5)

% Since we know we will be moving the deltaP depends on how the hoses are
% conneted, and so we put absolute value on it do be sure.

dP = 5000*(ADC/Vs - 0.5);
dP = abs(dP);

airspeed = sqrt(2*dP/rho);

== matlab function VTOL_v2/Subsystem1/MATLAB Function ==
  data: t input single size=1; r output single size=1; p output single size=1
function [r, p] = fcn(t)

t1 = 1;
t2 = 2;
t3 = 3;
t4 = 4;
t5 = 6;
t6 = 7;
t7 = 8;
t8 = 9;
r = single(0);
p = single(0);

if t<t1
    r = single(0);
    p = single(0);
elseif t<t2
    r = single(1);
    p = single(0);
elseif t<t3
    r = single(0);
    p = single(0);
elseif t<t4
    r = single(-1);
    p = single(0);
elseif t<t5
    r = single(0);
    p = single(0);
elseif t<t6
    r = single(0);
    p = single(1);
elseif t<t7
    r = single(0);
    p = single(0);
 elseif t<t8
    r = single(0);
    p = single(-1);
else % Safeguard
    r = single(0);
    p = single(0);
end

== matlab function VTOL_v2/Subsystem1/MATLAB Function17 ==
  data: y output single; en input boolean; in input single
function y = hardon(en, in)
%At first arm, start logging and dont quit

persistent state;
persistent hold;

if isempty(state)
    state = single(0);
end
if isempty(hold)
    hold = single(0);
end

if en>0 && hold==0
    state = in;
    hold=single(1);
end

y = state;

== matlab function VTOL_v2/MATLAB Function1 ==
  data: sats input; gps_good output; hdop input; vdop input
function gps_good = fcn(sats, hdop, vdop)

gps_good = single(0);

if sats > 5 && abs(hdop-1) < 2 && abs(vdop-1) < 2
    gps_good = single(1);
else
    gps_good = single(0);
end
